simulink model "sampleModel1866_3_sub_sub"  (R2023a)
settings: Solver=VariableStepAuto  StartTime=0.0  StopTime=10.0  RelTol=1e-3
libraries: hdlsllib x2, simulink x1
settings Model: Creator=user1  LastModifiedBy=user1
settings OptimizationCC: BlockReduction=off  ConditionallyExecuteInputs=off

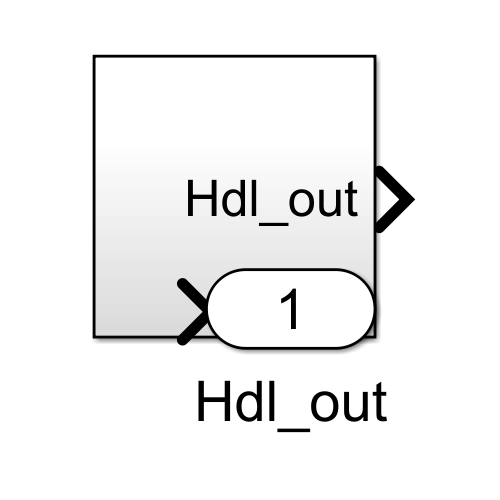
[thumbnail: Simulink's stored preview of the top-level diagram]
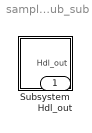
== system sampleModel1866_3_sub_sub ==
  Subsystem : Subsystem
  Hdl_out : Outport  OutDataTypeStr=uint8

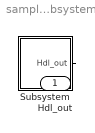
== system sampleModel1866_3_sub_sub/Subsystem ==
  Subsystem : Subsystem
  Hdl_out : Outport  OutDataTypeStr=uint8
  wires:
  Subsystem/1(Hdl_out) -> Hdl_out/1

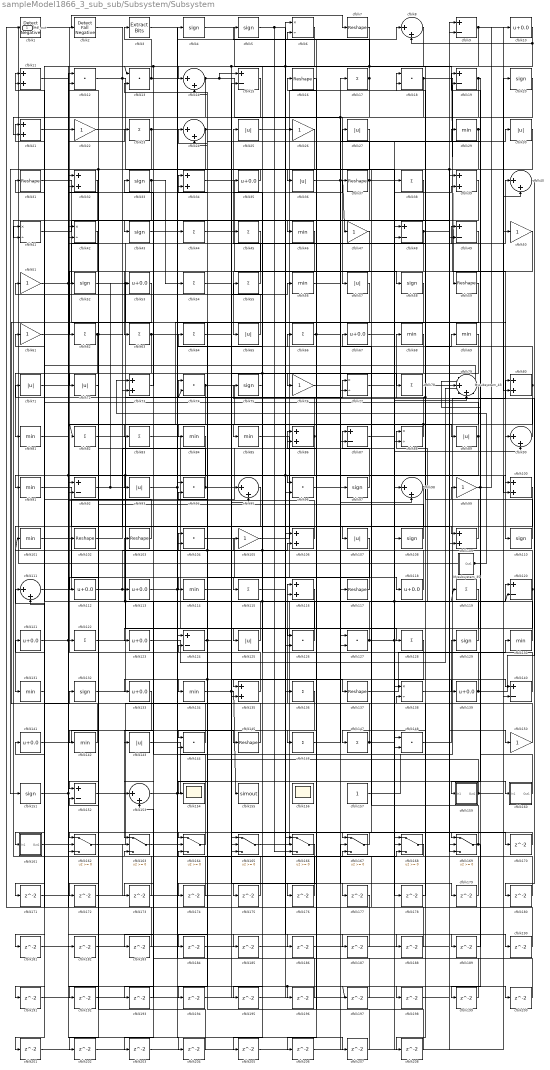
== system sampleModel1866_3_sub_sub/Subsystem/Subsystem ==
  Mysubsystem_35 : Subsystem  TreatAsAtomicUnit=on  RTWFcnName=Mysubsystem_35
      settings: RTWFcnNameOpts=User specified  RTWFileNameOpts=Use function name
  Mysubsystem_43 : Subsystem  TreatAsAtomicUnit=on  RTWFcnName=Mysubsystem_43
      settings: RTWFcnNameOpts=User specified  RTWFileNameOpts=Use function name
  cfblk1 : hdlsllib/Logic and Bit Operations/Detect Fall Negative  vinit=0  OutDataTypeStr=uint8
  cfblk{10,35,53,67,112..113,118,121,123,133,139,141} (12 alike) : Bias  Bias=0.0  SaturateOnIntegerOverflow=off
  cfblk{11,21,32,34,39,73,80,86,100,106,109,116,135} (13 alike) : Sum  OutDataTypeStr=uint8
  cfblk{29,46,56,68..69,81,84..85,91,101,114,130..131,134,142} (15 alike) : MinMax  OutDataTypeStr=uint8
  cfblk{7,16,31,37,59,102..103,117,137,145} (10 alike) : Reshape
  cfblk{12..13,18,74,94,96,104,126..127,144,148} (11 alike) : DotProduct  OutDataTypeStr=uint8
  cfblk{22,26,47,50..51,61,76,99,105,150} (10 alike) : Gain  OutDataTypeStr=uint8
  cfblk{25,27,30,36,57,65,71..72,89,93,107,125,143} (13 alike) : Abs  OutDataTypeStr=uint8  SaturateOnIntegerOverflow=off
  cfblk{4..5,20,33,43,52,58,75,97,108,110,129,132,151} (14 alike) : Signum
  cfblk{8,14,24,40,79,90,95,98,111,153} (10 alike) : Sum  Inputs=|++  OutDataTypeStr=uint8
  cfblk{17,23,38,44..45,54..55,62..64,66,78,82..83,115,119,122,128,136,146..147} (21 alike) : Sum  Inputs=+  OutDataTypeStr=uint8
  cfblk{9,15,19,48..49,87,92,120,124,140,152} (11 alike) : Sum  Inputs=+-  OutDataTypeStr=uint8
  cfblk{6,41..42,77,88,138} (6 alike) : Product  Inputs=*/  OutDataTypeStr=uint8  RndMeth=Zero  SaturateOnIntegerOverflow=on
  cfblk154 : Scope
  cfblk155 : ToWorkspace  VariableName=simout  SaveFormat=Timeseries  SampleTime=-1
  cfblk156 : Scope
      settings: Floating=on
  cfblk157 : Constant  OutDataTypeStr=uint8  SampleTime=-1
  cfblk159 : Subsystem
      settings: LibrarySourceBlock=|
      | hdlsllib/Ports &
      | Subsystems/Subsystem
  cfblk160 : Subsystem
      settings: LibrarySourceBlock=|
      | hdlsllib/Ports &
      | Subsystems/Subsystem
  cfblk161 : Subsystem
      settings: LibrarySourceBlock=|
      | hdlsllib/Ports &
      | Subsystems/Subsystem
  cfblk{162..169} (8 alike) : Switch  OutDataTypeStr=uint8  SaturateOnIntegerOverflow=off  InputSameDT=off
  cfblk{170..208} (39 alike) : Delay  SampleTime=1
  cfblk2 : hdlsllib/Logic and Bit Operations/Detect Fall Negative  vinit=0  OutDataTypeStr=uint8
  cfblk3 : simulink/Logic and Bit Operations/Extract Bits  bitsToExtract=Upper half  numBits=8  bitIdxRange=[0 7]  outScalingMode=Preserve fixed-point scaling
      settings: LibrarySourceBlock=|
      | hdlsllib/Logic and Bit
      | Operations/Extract Bits
  Hdl_out : Outport  OutDataTypeStr=uint8
  wires:
  Mysubsystem_43/1(Out1) -> cfblk181/1
  cfblk123/1 -> Mysubsystem_43/2(In2)
  Mysubsystem_35/1(Out1) -> cfblk73/1, Hdl_out/1
  cfblk208/1 -> cfblk164/3
  cfblk207/1 -> cfblk86/2
  cfblk206/1 -> cfblk9/2
  cfblk16/1 -> cfblk206/1
  cfblk205/1 -> cfblk167/2
  cfblk204/1 -> cfblk152/2
  cfblk203/1 -> cfblk148/2
  cfblk84/1 -> cfblk203/1
  cfblk202/1 -> cfblk140/2
  cfblk201/1 -> cfblk168/1
  cfblk200/1 -> cfblk124/1
  cfblk81/1 -> cfblk200/1
  cfblk199/1 -> cfblk14/2
  cfblk198/1 -> cfblk39/1
  cfblk197/1 -> cfblk163/3
  cfblk196/1 -> cfblk34/2
  cfblk195/1 -> cfblk106/1
  cfblk194/1 -> cfblk6/1
  cfblk166/1 -> cfblk194/1
  cfblk193/1 -> cfblk153/2
  cfblk192/1 -> cfblk165/2
  cfblk191/1 -> cfblk48/2
  cfblk190/1 -> cfblk167/3
  cfblk189/1 -> cfblk19/2
  cfblk161/1(Out1) -> cfblk189/1
  cfblk188/1 -> cfblk12/1
  cfblk187/1 -> cfblk32/2
  cfblk186/1 -> cfblk88/2
  cfblk185/1 -> cfblk168/2
  cfblk3/1 -> cfblk185/1
  cfblk184/1 -> cfblk126/2
  cfblk57/1 -> cfblk184/1
  cfblk183/1 -> cfblk111/2
  cfblk182/1 -> cfblk79/1
  cfblk11/1 -> cfblk182/1
  cfblk181/1 -> cfblk95/1
  cfblk180/1 -> cfblk94/1
  cfblk40/1 -> cfblk180/1
  cfblk179/1 -> cfblk24/2
  cfblk178/1 -> cfblk138/2
  cfblk87/1 -> cfblk178/1
  cfblk177/1 -> cfblk1/1
  cfblk176/1 -> cfblk104/2
  cfblk49/1 -> cfblk176/1
  cfblk175/1 -> cfblk41/1
  cfblk30/1 -> cfblk175/1
  cfblk174/1 -> cfblk164/2
  cfblk119/1 -> cfblk174/1
  cfblk173/1 -> cfblk162/2
  cfblk116/1 -> cfblk173/1
  cfblk172/1 -> cfblk163/2
  cfblk50/1 -> cfblk172/1
  cfblk171/1 -> cfblk15/2
  cfblk170/1 -> cfblk162/1
  cfblk115/1 -> cfblk170/1
  cfblk19/1 -> cfblk159/1(In1), cfblk21/2
  cfblk37/1 -> cfblk139/1, cfblk13/2, cfblk195/1
  cfblk114/1 -> cfblk56/1
  cfblk151/1 -> cfblk23/1, cfblk188/1
  cfblk25/1 -> cfblk26/1
  cfblk86/1 -> cfblk34/1, cfblk123/1
  cfblk79/1 -> cfblk143/1
  cfblk163/1 -> cfblk168/3
  cfblk150/1 -> cfblk94/2
  cfblk100/1 -> cfblk112/1
  cfblk6/1 -> cfblk153/1, cfblk91/1
  cfblk124/1 -> cfblk104/1, cfblk169/2
  cfblk78/1 -> cfblk150/1
  cfblk91/1 -> cfblk166/1
  cfblk23/1 -> cfblk142/1, cfblk198/1
  cfblk93/1 -> cfblk66/1, cfblk207/1
  cfblk64/1 -> cfblk89/1
  cfblk51/1 -> cfblk20/1, cfblk84/1
  cfblk99/1 -> cfblk19/1, cfblk10/1
  cfblk148/1 -> cfblk129/1
  cfblk121/1 -> cfblk196/1, cfblk197/1, cfblk37/1
  cfblk80/1 -> cfblk18/2, cfblk109/1
  cfblk46/1 -> cfblk63/1
  cfblk15/1 -> cfblk162/3
  cfblk9/1 -> cfblk80/2, cfblk208/1
  cfblk110/1 -> cfblk99/1
  cfblk136/1 -> cfblk144/1
  cfblk85/1 -> cfblk148/1
  cfblk102/1 -> cfblk86/1
  cfblk8/1 -> cfblk42/2, cfblk165/3
  cfblk129/1 -> cfblk24/1
  cfblk118/1 -> cfblk35/1, cfblk11/2
  cfblk75/1 -> cfblk135/1
  cfblk108/1 -> cfblk42/1
  cfblk88/1 -> cfblk11/1, cfblk82/1
  cfblk133/1 -> cfblk163/1
  cfblk144/1 -> cfblk122/1
  cfblk104/1 -> cfblk127/1
  cfblk62/1 -> cfblk109/2, cfblk202/1, cfblk201/1
  cfblk67/1 -> cfblk79/2
  cfblk27/1 -> cfblk126/1
  cfblk34/1 -> cfblk138/1
  cfblk159/1(Out1) -> cfblk50/1, cfblk124/2
  cfblk2/1 -> cfblk49/2
  cfblk76/1 -> cfblk49/1
  cfblk44/1 -> cfblk58/1
  cfblk24/1 -> cfblk72/1, cfblk92/2, cfblk77/2
  cfblk5/1 -> cfblk100/2, cfblk187/1, cfblk166/3
  cfblk48/1 -> cfblk9/1, cfblk166/2
  cfblk52/1 -> cfblk38/1, cfblk144/2
  cfblk39/1 -> cfblk73/2
  cfblk169/1 -> cfblk67/1, cfblk199/1
  cfblk160/1(Out1) -> cfblk27/1
  cfblk21/1 -> cfblk96/2, cfblk204/1
  cfblk96/1 -> cfblk29/1
  cfblk138/1 -> cfblk140/1
  cfblk164/1 -> cfblk113/1
  cfblk157/1 -> cfblk80/1
  cfblk66/1 -> cfblk16/1, cfblk100/1
  cfblk126/1 -> cfblk61/1, cfblk105/1
  cfblk141/1 -> cfblk145/1
  cfblk90/1 -> cfblk75/1
  cfblk61/1 -> cfblk102/1
  cfblk109/1 -> cfblk74/2, cfblk45/1
  cfblk94/1 -> cfblk12/2, cfblk177/1
  cfblk43/1 -> cfblk4/1
  cfblk12/1 -> cfblk36/1, cfblk96/1
  cfblk137/1 -> cfblk40/2
  cfblk128/1 -> cfblk154/1, cfblk183/1
  cfblk77/1 -> cfblk90/2
  cfblk153/1 -> cfblk120/1, cfblk190/1
  cfblk56/1 -> cfblk98/2
  cfblk120/1 -> cfblk74/1, cfblk101/1, cfblk193/1
  cfblk54/1 -> cfblk78/1
  cfblk72/1 -> cfblk152/1
  cfblk127/1 -> cfblk39/2, cfblk120/2, cfblk169/1, cfblk103/1
  cfblk162/1 -> cfblk44/1
  cfblk152/1 -> cfblk95/2
  cfblk131/1 -> cfblk111/1
  cfblk74/1 -> cfblk117/1, cfblk192/1
  cfblk22/1 -> cfblk98/1
  cfblk31/1 -> cfblk90/1
  cfblk10/1 -> cfblk8/2, cfblk205/1
  cfblk103/1 -> cfblk71/1
  cfblk147/1 -> cfblk119/1, cfblk30/1, cfblk116/2
  cfblk167/1 -> cfblk164/1
  cfblk140/1 -> cfblk55/1
  cfblk122/1 -> cfblk77/1, cfblk108/1
  cfblk125/1 -> cfblk21/1
  cfblk89/1 -> cfblk31/1, cfblk191/1
  cfblk146/1 -> cfblk97/1
  cfblk145/1 -> cfblk32/1
  cfblk113/1 -> cfblk69/1, cfblk160/1(In1)
  cfblk97/1 -> cfblk87/1
  cfblk68/1 -> cfblk161/1(In1)
  cfblk112/1 -> cfblk40/1, cfblk106/2
  cfblk20/1 -> cfblk76/1, cfblk87/2
  cfblk168/1 -> cfblk141/1
  cfblk13/1 -> cfblk3/1, cfblk186/1
  cfblk130/1 -> cfblk88/1
  cfblk32/1 -> cfblk41/2
  cfblk42/1 -> cfblk62/1
  cfblk26/1 -> cfblk133/1
  cfblk18/1 -> cfblk110/1, cfblk93/1
  cfblk47/1 -> cfblk146/1
  cfblk71/1 -> cfblk22/1
  cfblk4/1 -> cfblk59/1, cfblk136/1
  cfblk111/1 -> cfblk48/1
  cfblk134/1 -> cfblk155/1, cfblk137/1
  cfblk63/1 -> cfblk81/1, cfblk8/1
  cfblk69/1 -> cfblk115/1, cfblk171/1
  cfblk38/1 -> cfblk46/1
  cfblk73/1 -> cfblk33/1
  cfblk106/1 -> cfblk92/1
  cfblk7/1 -> cfblk14/1
  cfblk139/1 -> cfblk68/1, cfblk6/2
  cfblk14/1 -> cfblk15/1, cfblk127/2, cfblk83/1
  cfblk55/1 -> cfblk25/1
  cfblk107/1 -> cfblk134/1
  cfblk165/1 -> cfblk17/1
  cfblk36/1 -> cfblk47/1, cfblk179/1
  cfblk65/1 -> cfblk51/1
  cfblk29/1 -> Mysubsystem_43/1(In1), cfblk107/1, cfblk169/3
  cfblk135/1 -> cfblk2/1
  cfblk58/1 -> cfblk167/1
  cfblk35/1 -> cfblk151/1
  cfblk17/1 -> cfblk13/1, cfblk5/1, cfblk57/1
  cfblk101/1 -> cfblk114/1
  cfblk143/1 -> cfblk130/1
  cfblk142/1 -> cfblk121/1
  cfblk132/1 -> cfblk116/1
  cfblk45/1 -> cfblk65/1
  cfblk105/1 -> cfblk18/1
  cfblk59/1 -> cfblk85/1
  cfblk41/1 -> cfblk43/1
  cfblk83/1 -> cfblk125/1
  cfblk92/1 -> cfblk118/1, cfblk53/1
  cfblk98/1 -> cfblk147/1, cfblk135/2
  cfblk33/1 -> cfblk54/1, cfblk52/1
  cfblk53/1 -> cfblk132/1
  cfblk82/1 -> cfblk128/1, cfblk165/1
  cfblk117/1 -> cfblk64/1
  cfblk1/1 -> cfblk7/1
  cfblk95/1 -> cfblk131/1

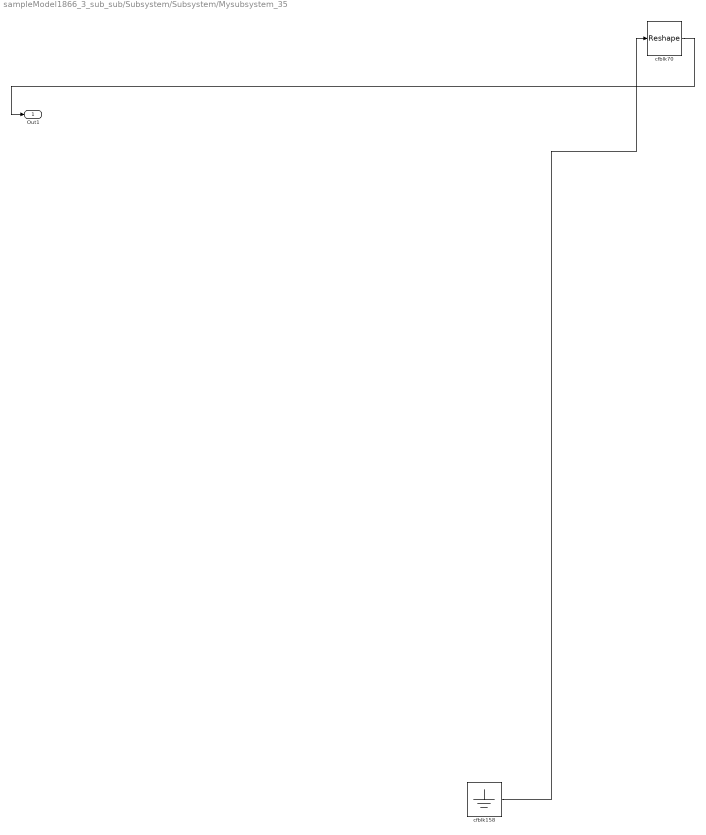
== system sampleModel1866_3_sub_sub/Subsystem/Subsystem/Mysubsystem_35 ==
  cfblk158 : Ground
  cfblk70 : Reshape
  Out1 : Outport
  wires:
  cfblk158/1 -> cfblk70/1
  cfblk70/1 -> Out1/1

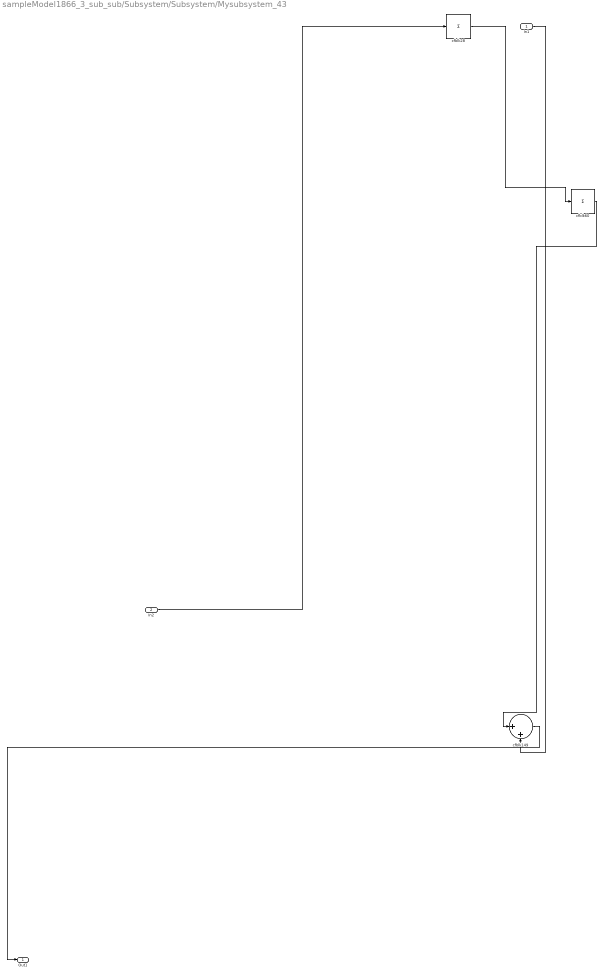
== system sampleModel1866_3_sub_sub/Subsystem/Subsystem/Mysubsystem_43 ==
  In1 : Inport
  In2 : Inport  Port=2
  cfblk149 : Sum  Inputs=|++
  cfblk28 : Sum  Inputs=+
  cfblk60 : Sum  Inputs=+
  Out1 : Outport
  wires:
  cfblk60/1 -> cfblk149/1
  cfblk28/1 -> cfblk60/1
  In1/1 -> cfblk149/2
  In2/1 -> cfblk28/1
  cfblk149/1 -> Out1/1

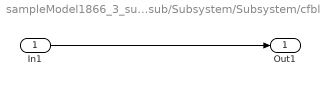
== system sampleModel1866_3_sub_sub/Subsystem/Subsystem/cfblk159 ==
  In1 : Inport
  Out1 : Outport
  wires:
  In1/1 -> Out1/1

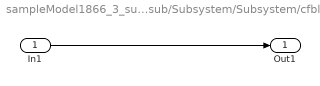
== system sampleModel1866_3_sub_sub/Subsystem/Subsystem/cfblk160 ==
  In1 : Inport
  Out1 : Outport
  wires:
  In1/1 -> Out1/1

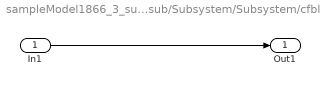
== system sampleModel1866_3_sub_sub/Subsystem/Subsystem/cfblk161 ==
  In1 : Inport
  Out1 : Outport
  wires:
  In1/1 -> Out1/1
